simulink model "contenedor_hegaps"  (R2020b)
settings: Solver=VariableStepAuto  StartTime=0.0  StopTime=0.3  RelTol=1e-3
InitFcn:
  | Ts=100e-6;
StartFcn:
  | Ts=100e-6;
libraries: powerlib x10
settings Model: Creator=JGC  LastModifiedBy=JGC
settings DataIOCC: ReturnWorkspaceOutputs=off

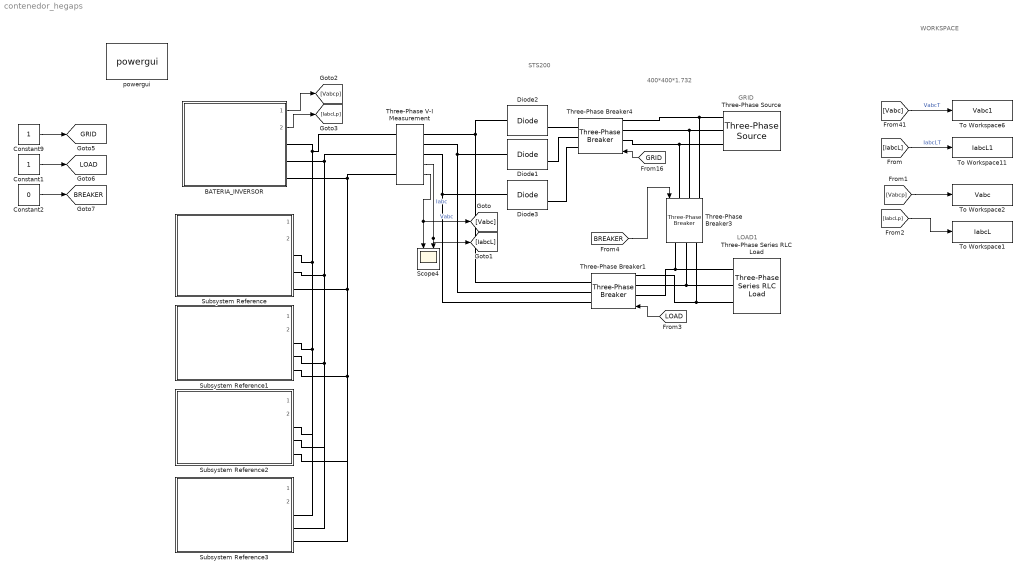
== system contenedor_hegaps ==
  note: STS200
  note: LOAD1
  note: GRID
  note: 400*400*1.732
  note: WORKSPACE
  BATERIA_INVERSOR : Subsystem  ReferencedSubsystem=BATERIA_INVERSOR
  Constant1 : Constant
  Constant2 : Constant  Value=0
  Constant9 : Constant
  Diode1 : powerlib/Power Electronics/Diode  Ron=0.001  Lon=0  Vf=0.8  IC=0  UseSnubber=0  Rs=500  Cs=250e-9  Measurements=on
  Diode2 : powerlib/Power Electronics/Diode  Ron=0.001  Lon=0  Vf=0.8  IC=0  UseSnubber=0  Rs=500  Cs=250e-9  Measurements=on
  Diode3 : powerlib/Power Electronics/Diode  Ron=0.001  Lon=0  Vf=0.8  IC=0  UseSnubber=0  Rs=500  Cs=250e-9  Measurements=on
  Scope4 : Scope  NumInputPorts=2
  Subsystem Reference{,1..3} (4 alike) : Subsystem  ReferencedSubsystem=BATERIA_INVERSOR
  Three-Phase Series RLC Load : powerlib/Elements/Three-Phase Series RLC Load  LConnTagsString=A|B|C  Configuration=Y (grounded)  NominalVoltage=400  Vabc=[1e3 1e3 1e3]  Vabcp=[1e3 1e3 1e3]  NominalFrequency=50  UnbalancedPower=off  ActivePower=250e3  InductivePower=100  CapacitivePower=100  Pabc=[10e3 9e3 11e3]  QLabc=[100 90 110]  QCabc=[100 90 110]  Pabcp=[10e3 9e3 11e3]  QLabcp=[100 90 110]  QCabcp=[100 90 110]  Measurements=None  LoadType=constant Z
  Three-Phase V-I Measurement : powerlib/Measurements/Three-Phase V-I Measurement  VoltageMeasurement=phase-to-phase  SetLabelV=off  LabelV=Vabc  Vpu=off  VpuLL=off  CurrentMeasurement=yes  SetLabelI=off  LabelI=Iabc  Ipu=off  Pbase=100e6  Vbase=500e3  OutputType=Complex  PhasorSimulation=off  PSBequivalent=0
  Three-Phase Breaker1 : powerlib/Elements/Three-Phase Breaker  InitialState=closed  SwitchA=on  SwitchB=on  SwitchC=on  SwitchTimes="[1/60  5/60]"  External=on  BreakerResistance=0.01  SnubberResistance=1e6  SnubberCapacitance=inf  Measurements=None
  Three-Phase Breaker3 : powerlib/Elements/Three-Phase Breaker  InitialState=closed  SwitchA=on  SwitchB=on  SwitchC=on  SwitchTimes="[1/60  5/60]"  External=on  BreakerResistance=0.01  SnubberResistance=1e6  SnubberCapacitance=inf  Measurements=None
  Three-Phase Breaker4 : powerlib/Elements/Three-Phase Breaker  InitialState=closed  SwitchA=on  SwitchB=on  SwitchC=on  SwitchTimes="[1/60  5/60]"  External=on  BreakerResistance=0.01  SnubberResistance=1e6  SnubberCapacitance=inf  Measurements=None
  Three-Phase Source : powerlib/Electrical Sources/Three-Phase Source  InternalConnection=Y  VoltagePhases=off  Voltage=400  PhaseAngle=0  Voltage_phases=[25e3 25e3 25e3]/sqrt(3)  PhaseAngles_phases=[0 -120 +120]  Frequency=50  NonIdealSource=on  SpecifyImpedance=off  Resistance=0.0001e-3  Inductance=0.0001e-9  ShortCircuitLevel=100e6  BaseVoltage=400  XRratio=7  BusType=swing  Pref=10e3  Qref=0  Prefabc=[10e3, 10e3, 10e3]  Qrefabc=[0, 0, 0]  Qmin=-inf  Qmax=inf
  To Workspace1 : ToWorkspace  VariableName=IabcL  SaveFormat=Structure With Time  SampleTime=-1
  To Workspace11 : ToWorkspace  VariableName=IabcL1  SaveFormat=Structure With Time  SampleTime=-1
  To Workspace2 : ToWorkspace  VariableName=Vabc  SaveFormat=Structure With Time  SampleTime=-1
  To Workspace6 : ToWorkspace  VariableName=Vabc1  SaveFormat=Structure With Time  SampleTime=-1
  powergui : powerlib/powergui  Priority=1  SimulationMode=Discrete  SampleTime=1e-5  frequency=60  Iterations=50  frequencyindice=0  Pbase=100e6  ErrMax=1e-4  UnitsV=kV  UnitsW=MW  buscounter=0  FunctionMessages=off  echomessages=off  EnableUseOfTLC=off  CurrentSourceSwitches=off  DisableSnubberDevices=off  DisableRonSwitches=off  DisableVfSwitches=off  DisplayEquations=off  AutomaticDiscreteSolvers=off  SolverType=Tustin/Backward Euler (TBE)  Interpol=off  ExternalGateDelay=off  methode=off  Ts=100  x0status=blocks  SPID=on  SwTol=0  HookPort=off  NonlinearTolerance=1e-4  nMaxIteration=100  ContinueOnMaxIteration=off  RestoreLinks=warning  ResistiveCurrentMeasurement=off  Frange=[0:2:500]  Ylog=off  Xlog=on  ShowGrid=off  save=off  variable=ZData  structure=IabcL1  ZoomFFT=off  StartTime=0.03  cycles=9  DisplayStyle=1  fundamental=50  FreqAxis=off  MaxFrequency=10000  frequencyindicesteady=1  RmsSteady=1  display=off
  tag scope: BREAKER=global, GRID=global, LOAD=global
  wires:
  Constant9/1 -> [GRID]
  [GRID] -> Three-Phase Breaker4/1
  [LOAD] -> Three-Phase Breaker1/1
  [BREAKER] -> Three-Phase Breaker3/1
  Constant1/1 -> [LOAD]
  Constant2/1 -> [BREAKER]
  Three-Phase V-I Measurement/1 -> [Vabc], Scope4/1  "Vabc"
  Three-Phase V-I Measurement/2 -> [IabcL], Scope4/2  "Iabc"
  [IabcL] -> To Workspace11/1  "IabcLT"
  [Vabc] -> To Workspace6/1  "VabcT"
  [Vabcp] -> To Workspace2/1
  [IabcLp] -> To Workspace1/1
  BATERIA_INVERSOR/1 -> [Vabcp]
  BATERIA_INVERSOR/2 -> [IabcLp]
  connections:
  Three-Phase Source/RConn1 -- Three-Phase Breaker4/LConn1 -- Three-Phase Breaker3/LConn1
  Three-Phase Source/RConn2 -- Three-Phase Breaker4/LConn2 -- Three-Phase Breaker3/LConn2
  Diode2/LConn1 -- Three-Phase V-I Measurement/RConn3 -- Three-Phase Breaker1/RConn3
  Three-Phase Source/RConn3 -- Three-Phase Breaker4/LConn3 -- Three-Phase Breaker3/LConn3
  Diode1/LConn1 -- Three-Phase V-I Measurement/RConn2 -- Three-Phase Breaker1/RConn2
  Diode3/LConn1 -- Three-Phase V-I Measurement/RConn1 -- Three-Phase Breaker1/RConn1
  Three-Phase Breaker1/LConn3 -- Three-Phase Breaker3/RConn3 -- Three-Phase Series RLC Load/LConn3
  Three-Phase Breaker1/LConn2 -- Three-Phase Breaker3/RConn2 -- Three-Phase Series RLC Load/LConn2
  Three-Phase Breaker1/LConn1 -- Three-Phase Breaker3/RConn1 -- Three-Phase Series RLC Load/LConn1
  Diode2/RConn1 -- Three-Phase Breaker4/RConn3
  Diode1/RConn1 -- Three-Phase Breaker4/RConn2
  Diode3/RConn1 -- Three-Phase Breaker4/RConn1
  BATERIA_INVERSOR/RConn3 -- Subsystem Reference3/RConn3 -- Subsystem Reference2/RConn3 -- Subsystem Reference1/RConn3 -- Subsystem Reference/RConn3 -- Three-Phase V-I Measurement/LConn1
  Three-Phase V-I Measurement/LConn2 -- Subsystem Reference3/RConn2 -- Subsystem Reference2/RConn2 -- Subsystem Reference1/RConn2 -- Subsystem Reference/RConn2 -- BATERIA_INVERSOR/RConn2
  BATERIA_INVERSOR/RConn1 -- Subsystem Reference3/RConn1 -- Subsystem Reference2/RConn1 -- Subsystem Reference1/RConn1 -- Subsystem Reference/RConn1 -- Three-Phase V-I Measurement/LConn3
